simulink model "a1_euler"  (Simulink 8.7)
settings: Solver=VariableStepAuto  StartTime=0.0  StopTime=0.2  FixedStep=0.005  RelTol=1e-3
libraries: simulink x1
settings Model: Creator=birger  LastModifiedBy=birger
settings DataIOCC: LimitDataPoints=off  SaveFormat=Dataset
settings DebuggingCC: UnderspecifiedInitializationDetection=Simplified  MergeDetectMultiDrivingBlocksExec=error
settings HardwareCC: ProdBitPerPointer=64  ProdLargestAtomicFloat=Float  ProdIntDivRoundTo=Zero  ProdEndianess=LittleEndian  ProdWordSize=64  ProdHWDeviceType=Intel->x86-64 (Windows64)
settings ModelReferenceCC: PropagateSignalLabelsOutOfModel=on
settings ConfigComp: CovModelRefEnable=off

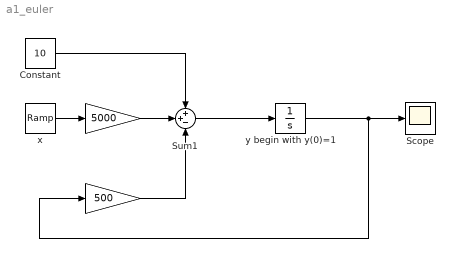
== system a1_euler ==
  " " : Gain  Gain=500
  "  " : Gain  Gain=5000
  Constant : Constant  Value=10
  Scope : Scope
  Sum1 : Sum  Inputs=++-
  x : simulink/Sources/Ramp  slope=1  start=0  X0=0
  y begin with y(0)=1 : Integrator  InitialCondition=1
  wires:
  Constant/1 -> Sum1/1
  x/1 -> "  "/1
  Sum1/1 -> y begin with y(0)=1/1
  y begin with y(0)=1/1 -> " "/1, Scope/1
  "  "/1 -> Sum1/2
  " "/1 -> Sum1/3
